simulink model "HEV_DCModel"  (R2019b)
settings: Solver=ode4  StartTime=0  StopTime=tEnd  FixedStep=dt  RelTol=1e-3
values from neighbouring files (symbols this model uses):
  accessoryLoad = 600    [main.m]
  Af = 1.00    (= 1)    [main.m]
  b = .002    (= 0.002)    [main.m]
  batteryCapacity = 50    [main.m]
  batteryResistance = 0.0461    [main.m]
  C = 400    [main.m]
  Cd = 0.576    [main.m]
  Crr = 0.01    [main.m]
  cycleNum = 2    [main.m]
  EffTableEff = [.75 .85 .89 .95 .96 .97 .98 .99 .99]    [main.m]
  EffTableSpeed = [0 5 10 15 25 35 45 55 65]    [main.m]
  etaGenGR = 0.93    [main.m]
  g = 9.81    [main.m]
  GRd = 9.843    [main.m]
  GRgen = 1.4    [main.m]
  initialGasVolume = 5    [main.m]
  Jm = 5    [main.m]
  k_gal2kWh = 32.3    [main.m]
  k_hr2s = 3600    [main.m]
  k_J2gal = 1/3600000/32.3    (= 8.59993120055e-09)    [main.m]
  k_kW2W = 1000    [main.m]
  k_kWh2J = 3.6*10^6    (= 3600000)    [main.m]
  k_m2mi = 0.000621371    [main.m]
  k_m32gal = 264.172    [main.m]
  k_rpm2rps = 2*pi()/60    [main.m]
  k_rps2rpm = 60/(2*pi)    (= 9.54929658551)    [main.m]
  k_s2h = 1/3600    (= 0.000277777777778)    [main.m]
  k_W2kW = 1/1000    (= 0.001)    [main.m]
  kc = 0.513    [main.m]
  Kd = 0    [main.m]
  KD_DC = 0    [main.m]
  ke = kt    (= 3)    [main.m]
  Ki = 0.1    [main.m]
  ki = 0.0773    [main.m]
  KI_DC = 0.1    [main.m]
  Kp = 200    [main.m]
  KP_DC = 200    [main.m]
  kt = 3    [main.m]
  kw = 0.0000064    (= 6.4e-06)    [main.m]
  La = .01    (= 0.01)    [main.m]
  m = 1965    [main.m]
  motorMaxPower = 310000    [main.m]
  motorMaxSpeed = 18000    [main.m]
  motorMaxTorque = 600    [main.m]
  openCircuitVoltage = 420    [main.m]
  pBrakeMax = 4*TbrakeMax / (mu_k*pi()* cylinderBore^2 *meanPadRadius*numPads)    [main.m]
  r = 0.290    (= 0.29)    [main.m]
  Ra = .06    (= 0.06)    [main.m]
  rho = 1.20    (= 1.2)    [main.m]
  SOCi = 90    [main.m]
  theta = 0    [main.m]
  v0 = 0    [main.m]
  x0 = 0    [main.m]
libraries: autolibshared x6, fl_lib x5, nesl_utility x5, sdl_lib x1, autolibsharedmappedengines x1, simulink x1
(part 3 of 3)

== system HEV_DCModel/DC Motor Genset/Gearbox ==
  Torque In [Nm] : Inport
  Power In [W] : Inport  Port=2
  Engine Speed [rad/s] : Inport  Port=3
  Add : Sum  Inputs=+-
  Bus Creator : BusCreator  Inputs=3
  Gain : Gain  Gain=GRgen
  Gain1 : Gain  Gain=k_W2kW
  Gain2 : Gain  Gain=etaGenGR
  Gain3 : Gain  Gain=1/GRgen
  Product1 : Product
  Torque Out [Nm] : Outport
  Info : Outport  Port=2
  wires:
  Gain2/1 -> [torqueOut], Torque Out [Nm]/1, Product1/1  "Torque Out [Nm]"
  Product1/1 -> Add/2  "Gearbox Power Out [W]"
  Engine Speed [rad/s]/1 -> Gain3/1
  Gain/1 -> Gain2/1
  Power In [W]/1 -> Add/1
  Add/1 -> Gain1/1  "Gearbox Power Loss [W]"
  Torque In [Nm]/1 -> [torqueIn], Gain/1
  Gain1/1 -> Bus Creator/1  "powerLoss"
  [torqueIn] -> Bus Creator/2  "torqueIn"
  [torqueOut] -> Bus Creator/3  "torqueOut"
  Bus Creator/1 -> Info/1  "gearbox"
  Gain3/1 -> Product1/2

== system HEV_DCModel/DC Motor Genset/Motor ==
  Engine Torque [Nm] : Inport
  Angular Velocity Command [rpm] : Inport  Port=2
  Motor Plant : Subsystem
  Motor Speed Controller : Subsystem
  Power Out [kW] : Outport
  Info : Outport  Port=2
  wires:
  Angular Velocity Command [rpm]/1 -> Motor Speed Controller/1(Angular Velocity Setpoint [rpm])
  Motor Speed Controller/1(Applied Voltage [V]) -> Motor Plant/2(Applied Voltage [V])
  Motor Plant/3(Angular Velocity [rad/s]) -> Motor Speed Controller/2(Angular Velocity [rad/s])
  Motor Plant/1(Info) -> Info/1
  Motor Plant/2(Power Out [kW]) -> Power Out [kW]/1
  Engine Torque [Nm]/1 -> Motor Plant/1(Engine Torque [Nm])

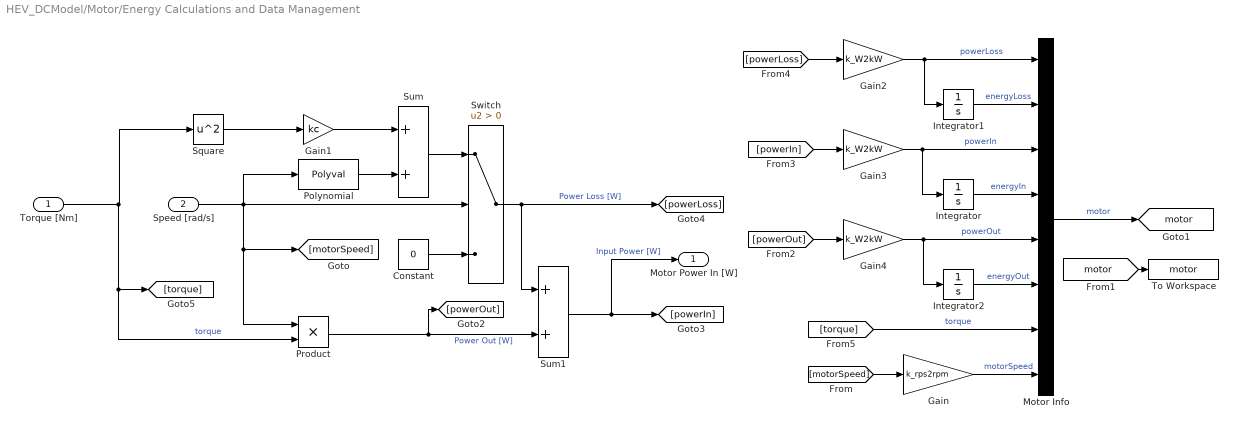
== system HEV_DCModel/Motor/Energy Calculations and Data Management ==
  Torque [Nm] : Inport
  Speed [rad/s] : Inport  Port=2
  Constant : Constant  Value=0
  Gain : Gain  Gain=k_rps2rpm
  Gain1 : Gain  Gain=kc
  Gain2 : Gain  Gain=k_W2kW
  Gain3 : Gain  Gain=k_W2kW
  Gain4 : Gain  Gain=k_W2kW
  Integrator : Integrator
  Integrator1 : Integrator
  Integrator2 : Integrator
  Motor Info : BusCreator  Inputs=8
  Polynomial : Polyval  Coefs=[kw , 0 ki, C]
  Product : Product
  Square : Math  Operator=square  SignedPower=off  SaturateOnIntegerOverflow=on
  Sum : Sum
  Sum1 : Sum
  Switch : Switch  Criteria=u2 > Threshold
  To Workspace : ToWorkspace  VariableName=motor  SaveFormat=Timeseries  SampleTime=-1
  Motor Power In [W] : Outport
  tag scope: motor=global
  wires:
  Motor Info/1 -> [motor]  "motor"
  Product/1 -> [powerOut], Sum1/2  "Power Out [W]"
  Speed [rad/s]/1 -> Polynomial/1, Product/1, [motorSpeed], Switch/2
  Constant/1 -> Switch/3
  Polynomial/1 -> Sum/2
  Sum/1 -> Switch/1
  Gain1/1 -> Sum/1
  Switch/1 -> Sum1/1, [powerLoss]  "Power Loss [W]"
  Sum1/1 -> Motor Power In [W]/1, [powerIn]  "Input Power [W]"
  Torque [Nm]/1 -> Square/1, Product/2, [torque]  "torque"
  Square/1 -> Gain1/1
  Integrator/1 -> Motor Info/4  "energyIn"
  Integrator2/1 -> Motor Info/6  "energyOut"
  Integrator1/1 -> Motor Info/2  "energyLoss"
  [motorSpeed] -> Gain/1
  Gain/1 -> Motor Info/8  "motorSpeed"
  [motor] -> To Workspace/1
  Gain4/1 -> Integrator2/1, Motor Info/5  "powerOut"
  Gain3/1 -> Motor Info/3, Integrator/1  "powerIn"
  Gain2/1 -> Motor Info/1, Integrator1/1  "powerLoss"
  [torque] -> Motor Info/7  "torque"
  [powerLoss] -> Gain2/1
  [powerIn] -> Gain3/1
  [powerOut] -> Gain4/1

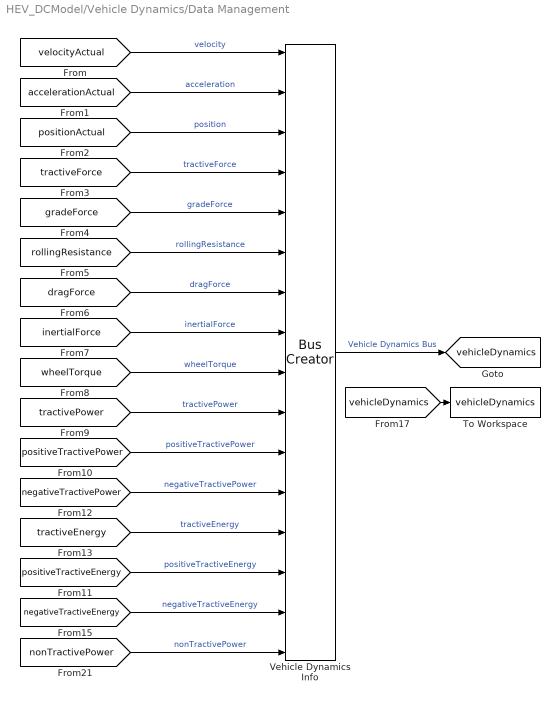
== system HEV_DCModel/Vehicle Dynamics/Data Management ==
  To Workspace : ToWorkspace  VariableName=vehicleDynamics  SaveFormat=Timeseries  SampleTime=-1
  Vehicle Dynamics Info : BusCreator  Inputs=16
  tag scope: vehicleDynamics=global
  wires:
  [velocityActual] -> Vehicle Dynamics Info/1  "velocity"
  [wheelTorque] -> Vehicle Dynamics Info/9  "wheelTorque"
  [tractiveForce] -> Vehicle Dynamics Info/4  "tractiveForce"
  [negativeTractivePower] -> Vehicle Dynamics Info/12  "negativeTractivePower"
  [accelerationActual] -> Vehicle Dynamics Info/2  "acceleration"
  [vehicleDynamics] -> To Workspace/1
  [gradeForce] -> Vehicle Dynamics Info/5  "gradeForce"
  [positiveTractivePower] -> Vehicle Dynamics Info/11  "positiveTractivePower"
  [positiveTractiveEnergy] -> Vehicle Dynamics Info/14  "positiveTractiveEnergy"
  [rollingResistance] -> Vehicle Dynamics Info/6  "rollingResistance"
  [inertialForce] -> Vehicle Dynamics Info/8  "inertialForce"
  [positionActual] -> Vehicle Dynamics Info/3  "position"
  [tractivePower] -> Vehicle Dynamics Info/10  "tractivePower"
  [negativeTractiveEnergy] -> Vehicle Dynamics Info/15  "negativeTractiveEnergy"
  [tractiveEnergy] -> Vehicle Dynamics Info/13  "tractiveEnergy"
  [dragForce] -> Vehicle Dynamics Info/7  "dragForce"
  [nonTractivePower] -> Vehicle Dynamics Info/16  "nonTractivePower"
  Vehicle Dynamics Info/1 -> [vehicleDynamics]  "Vehicle Dynamics Bus"

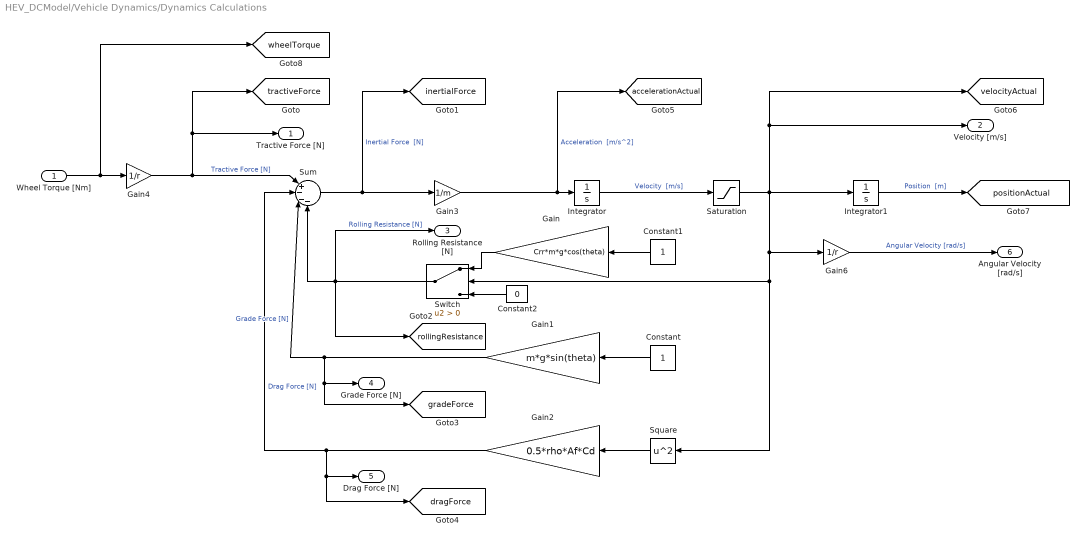
== system HEV_DCModel/Vehicle Dynamics/Dynamics Calculations ==
  Wheel Torque [Nm] : Inport
  Constant : Constant
  Constant1 : Constant
  Constant2 : Constant  Value=0
  Gain : Gain  Gain=Crr*m*g*cos(theta)
  Gain1 : Gain  Gain=m*g*sin(theta)
  Gain2 : Gain  Gain=0.5*rho*Af*Cd
  Gain3 : Gain  Gain=1/m
  Gain4 : Gain  Gain=1/r
  Gain6 : Gain  Gain=1/r
  Integrator : Integrator  InitialCondition=v0
  Integrator1 : Integrator  InitialCondition=x0
  Saturation : Saturate  UpperLimit=inf  LowerLimit=0  LinearizeAsGain=off
  Square : Math  Operator=square  SignedPower=off  SaturateOnIntegerOverflow=on
  Sum : Sum  Inputs=|+---
  Switch : Switch  Criteria=u2 > Threshold
  Tractive Force [N] : Outport
  Velocity [m/s] : Outport  Port=2
  Rolling Resistance [N] : Outport  Port=3
  Grade Force [N] : Outport  Port=4
  Drag Force [N] : Outport  Port=5
  Angular Velocity [rad/s] : Outport  Port=6
  tag scope: accelerationActual=global, dragForce=global, gradeForce=global, inertialForce=global, positionActual=global, rollingResistance=global, tractiveForce=global, velocityActual=global, wheelTorque=global
  wires:
  Gain1/1 -> Grade Force [N]/1, [gradeForce], Sum/3  "Grade Force [N]"
  Gain4/1 -> Tractive Force [N]/1, [tractiveForce], Sum/1  "Tractive Force [N]"
  Constant/1 -> Gain1/1
  Switch/1 -> Sum/4, [rollingResistance], Rolling Resistance [N]/1  "Rolling Resistance [N]"
  Integrator/1 -> Saturation/1  "Velocity  [m/s]"
  Integrator1/1 -> [positionActual]  "Position  [m]"
  Sum/1 -> [inertialForce], Gain3/1  "Inertial Force  [N]"
  Constant1/1 -> Gain/1
  Gain3/1 -> [accelerationActual], Integrator/1  "Acceleration  [m/s^2]"
  Gain2/1 -> Drag Force [N]/1, [dragForce], Sum/2  "Drag Force [N]"
  Wheel Torque [Nm]/1 -> [wheelTorque], Gain4/1
  Square/1 -> Gain2/1
  Saturation/1 -> Gain6/1, Square/1, Switch/2, Velocity [m/s]/1, [velocityActual], Integrator1/1
  Gain/1 -> Switch/1
  Constant2/1 -> Switch/3
  Gain6/1 -> Angular Velocity [rad/s]/1  "Angular Velocity [rad/s]"

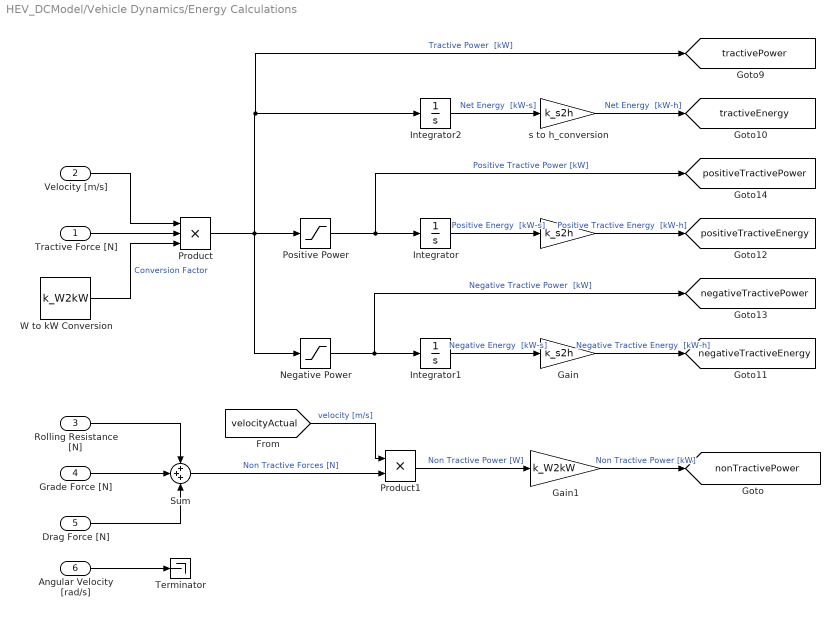
== system HEV_DCModel/Vehicle Dynamics/Energy Calculations ==
  Tractive Force [N] : Inport
  Velocity [m/s] : Inport  Port=2
  Rolling Resistance [N] : Inport  Port=3
  Grade Force [N] : Inport  Port=4
  Drag Force [N] : Inport  Port=5
  Angular Velocity [rad/s] : Inport  Port=6
  " " : Gain  Gain=k_s2h
  Gain : Gain  Gain=k_s2h
  Gain1 : Gain  Gain=k_W2kW
  Integrator : Integrator
  Integrator1 : Integrator
  Integrator2 : Integrator
  Negative Power : Saturate  UpperLimit=0  LowerLimit=-inf
  Positive Power : Saturate  UpperLimit=inf  LowerLimit=0
  Product : Product  Inputs=3
  Product1 : Product
  Sum : Sum  Inputs=+++
  Terminator : Terminator
  W to kW Conversion : Constant  Value=k_W2kW
  s to h_conversion : Gain  Gain=k_s2h
  tag scope: negativeTractiveEnergy=global, negativeTractivePower=global, nonTractivePower=global, positiveTractiveEnergy=global, positiveTractivePower=global, tractiveEnergy=global, tractivePower=global
  wires:
  s to h_conversion/1 -> [tractiveEnergy]  "Net Energy  [kW-h]"
  " "/1 -> [positiveTractiveEnergy]  "Positive Tractive Energy  [kW-h]"
  Gain/1 -> [negativeTractiveEnergy]  "Negative Tractive Energy  [kW-h]"
  Integrator1/1 -> Gain/1  "Negative Energy  [kW-s]"
  Integrator/1 -> " "/1  "Positive Energy  [kW-s]"
  Negative Power/1 -> [negativeTractivePower], Integrator1/1  "Negative Tractive Power  [kW]"
  Integrator2/1 -> s to h_conversion/1  "Net Energy  [kW-s]"
  Positive Power/1 -> [positiveTractivePower], Integrator/1  "Positive Tractive Power [kW]"
  W to kW Conversion/1 -> Product/3  "Conversion Factor"
  Product/1 -> Negative Power/1, [tractivePower], Integrator2/1, Positive Power/1  "Tractive Power  [kW]"
  Velocity [m/s]/1 -> Product/1
  Tractive Force [N]/1 -> Product/2
  Drag Force [N]/1 -> Sum/3
  Grade Force [N]/1 -> Sum/2
  Rolling Resistance [N]/1 -> Sum/1
  Sum/1 -> Product1/2  "Non Tractive Forces [N]"
  [velocityActual] -> Product1/1  "velocity [m/s]"
  Product1/1 -> Gain1/1  "Non Tractive Power [W]"
  Gain1/1 -> [nonTractivePower]  "Non Tractive Power [kW]"
  Angular Velocity [rad/s]/1 -> Terminator/1

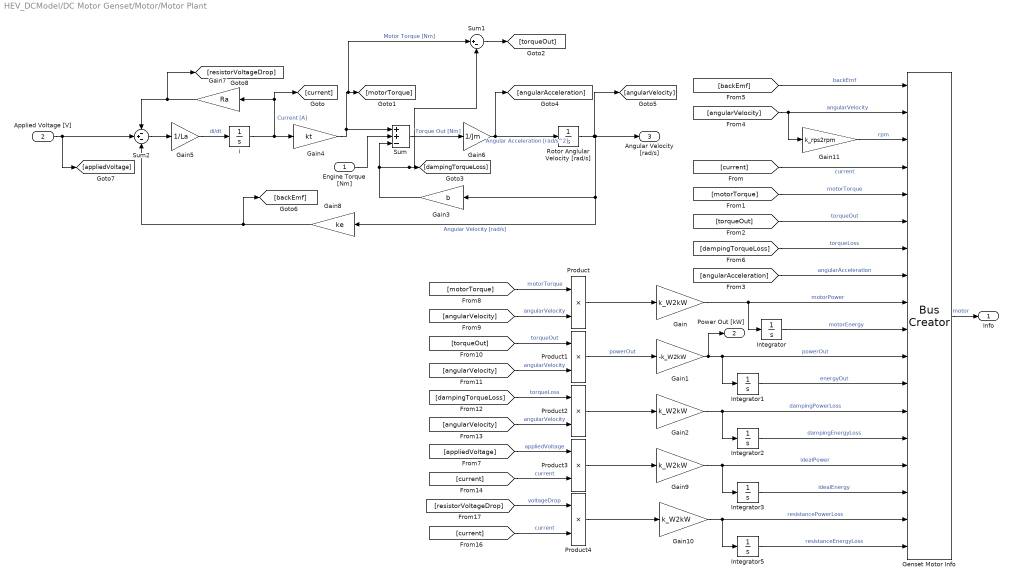
== system HEV_DCModel/DC Motor Genset/Motor/Motor Plant ==
  Engine Torque [Nm] : Inport
  Applied Voltage [V] : Inport  Port=2
  Gain{,2,9..10} (4 alike) : Gain  Gain=k_W2kW
  Gain1 : Gain  Gain=-k_W2kW
  Gain11 : Gain  Gain=k_rps2rpm
  Gain3 : Gain  Gain=b
  Gain4 : Gain  Gain=kt
  Gain5 : Gain  Gain=1/La
  Gain6 : Gain  Gain=1/Jm
  Gain7 : Gain  Gain=Ra
  Gain8 : Gain  Gain=ke
  Genset Motor Info : BusCreator  Inputs=18
  Integrator{,1..3,5} (5 alike) : Integrator
  Product{,1..4} (5 alike) : Product
  Rotor Anglular Velocity [rad/s] : Integrator
  Sum : Sum  Inputs=++-
  Sum1 : Sum  Inputs=|+-
  Sum2 : Sum  Inputs=-+-
  i : Integrator
  Info : Outport
  Power Out [kW] : Outport  Port=2
  Angular Velocity [rad/s] : Outport  Port=3
  wires:
  Sum/1 -> Gain6/1  "Torque Out [Nm]"
  Gain4/1 -> Sum1/1, [motorTorque], Sum/1  "Motor Torque [Nm]"
  Gain6/1 -> Rotor Anglular Velocity [rad/s]/1, [angularAcceleration]  "Angular Acceleration [rad/s^2]"
  i/1 -> Gain4/1, [current], Gain7/1  "Current [A]"
  Gain3/1 -> Sum/3, Sum1/2, [dampingTorqueLoss]
  Gain5/1 -> i/1  "di/dt"
  Rotor Anglular Velocity [rad/s]/1 -> Angular Velocity [rad/s]/1, Gain8/1, Gain3/1, [angularVelocity]  "Angular Velocity [rad/s]"
  Sum2/1 -> Gain5/1
  Applied Voltage [V]/1 -> Sum2/2, [appliedVoltage]
  Gain8/1 -> [backEmf], Sum2/3
  Gain7/1 -> [resistorVoltageDrop], Sum2/1
  Genset Motor Info/1 -> Info/1  "motor"
  Integrator2/1 -> Genset Motor Info/14  "dampingEnergyLoss"
  Gain10/1 -> Genset Motor Info/17, Integrator5/1  "resistancePowerLoss"
  Integrator3/1 -> Genset Motor Info/16  "idealEnergy"
  [torqueOut] -> Genset Motor Info/6  "torqueOut"
  [dampingTorqueLoss] -> Genset Motor Info/7  "torqueLoss"
  [torqueOut] -> Product1/1  "torqueOut"
  [appliedVoltage] -> Product3/1  "appliedVoltage"
  [angularVelocity] -> Product2/2  "angularVelocity"
  Integrator5/1 -> Genset Motor Info/18  "resistanceEnergyLoss"
  Product2/1 -> Gain2/1
  [angularAcceleration] -> Genset Motor Info/8  "angularAcceleration"
  Gain/1 -> Integrator/1, Genset Motor Info/9  "motorPower"
  Integrator1/1 -> Genset Motor Info/12  "energyOut"
  Product3/1 -> Gain9/1
  [angularVelocity] -> Product1/2  "angularVelocity"
  [current] -> Genset Motor Info/4  "current"
  Product/1 -> Gain/1
  Product1/1 -> Gain1/1  "powerOut"
  [current] -> Product3/2  "current"
  [backEmf] -> Genset Motor Info/1  "backEmf"
  [motorTorque] -> Genset Motor Info/5  "motorTorque"
  Gain11/1 -> Genset Motor Info/3  "rpm"
  [resistorVoltageDrop] -> Product4/1  "voltageDrop"
  [dampingTorqueLoss] -> Product2/1  "torqueLoss"
  Gain9/1 -> Genset Motor Info/15, Integrator3/1  "idealPower"
  Product4/1 -> Gain10/1
  Gain2/1 -> Integrator2/1, Genset Motor Info/13  "dampingPowerLoss"
  Integrator/1 -> Genset Motor Info/10  "motorEnergy"
  Gain1/1 -> Genset Motor Info/11, Integrator1/1, Power Out [kW]/1  "powerOut"
  [current] -> Product4/2  "current"
  [motorTorque] -> Product/1  "motorTorque"
  [angularVelocity] -> Gain11/1, Genset Motor Info/2  "angularVelocity"
  [angularVelocity] -> Product/2  "angularVelocity"
  Engine Torque [Nm]/1 -> Sum/2
  Sum1/1 -> [torqueOut]

== system HEV_DCModel/DC Motor Genset/Motor/Motor Speed Controller ==
  Angular Velocity Setpoint [rpm] : Inport
  Angular Velocity [rad/s] : Inport  Port=2
  Constant : Constant  Value=0
  Derivative : Derivative
  Gain10 : Gain  Gain=KI_DC
  Gain11 : Gain  Gain=KD_DC
  Gain12 : Gain  Gain=k_rpm2rps
  Gain9 : Gain  Gain=KP_DC
  Integrator3 : Integrator
  Saturation Dynamic : simulink/Discontinuities/Saturation Dynamic  OutMin=[]  OutMax=[]  OutDataTypeStr=Inherit: Same as second input  OutDataType=fixdt(1, 16)  OutScaling=2^-10  DoSatur=off
  Sum : Sum  Inputs=|+-
  Sum3 : Sum  Inputs=+++
  Applied Voltage [V] : Outport
  wires:
  Angular Velocity Setpoint [rpm]/1 -> Gain12/1
  Gain11/1 -> Derivative/1
  Integrator3/1 -> Sum3/2
  Sum/1 -> Gain11/1, Gain9/1, Gain10/1  "Error"
  Derivative/1 -> Sum3/3
  Gain10/1 -> Integrator3/1
  Gain9/1 -> Sum3/1
  Gain12/1 -> Sum/1  "Angular Velocity Setpoint [rad/s]"
  Angular Velocity [rad/s]/1 -> Sum/2
  Saturation Dynamic/1 -> Applied Voltage [V]/1  "Applied Voltage [V]"
  [busVoltage] -> Saturation Dynamic/1
  Constant/1 -> Saturation Dynamic/3
  Sum3/1 -> Saturation Dynamic/2

== stateflow chart HEV_DCModel/Thermostatic Hybrid Supervisory Controller /Chart ==
  state first
    entry:
    EngineTorque = 0;
    MotorSpeed = 0;
  state second
    entry:
    EngineTorque = 65;
    MotorSpeed = 800;
  (default) -> first
  first -> second : [FuelTankVolume > 0.2]
  second -> first : [FuelTankVolume < 0.2]
  data: SOC input; FuelTankVolume input; EngineTorque output; MotorSpeed output
